simulink model "CSTRExampleLinear"  (R2020a)
settings: Solver=FixedStepAuto  StartTime=0.0  StopTime=6  FixedStep=10e-3  MaxStep=10e-3  RelTol=1e-3
InitFcn:
  | CSTRInit;
values from neighbouring files (symbols this model uses):
  A = [-Fr0/V-k1-2*k3*Ca0, 0; k1, -Fr0/V-k2]    [CSTRInit.m]
  B = [6.341719*(Cai0-Ca0)/V, Fr0/V; -6.341719*Cb0/V, 0]    [CSTRInit.m]
  C = [0 100/1.5714]    [CSTRInit.m]
  Ca0 = 2.917496611031752    (= 2.91749661103)    [CSTRComputeOP.m]    (also in CSTRInit.m)
  Cai0 = 10    [CSTRInit.m]
  Cb0 = 1.099991103606458    (= 1.09999110361)    [CSTRComputeOP.m]    (also in CSTRInit.m)
  D = [0, 0]    [CSTRInit.m]
  k1 = 5/6    (= 0.833333333333)    [CSTRComputeOP.m]    (also in CSTRInit.m; CSTROP.m = param(1); sfun_CSTR.m = param(1))
  k2 = 5/3    (= 1.66666666667)    [CSTRComputeOP.m]    (also in CSTRInit.m; CSTROP.m = param(2); sfun_CSTR.m = param(2))
  k3 = 1/6    (= 0.166666666667)    [CSTRComputeOP.m]    (also in CSTRInit.m; CSTROP.m = param(3); sfun_CSTR.m = param(3))
  u0 = 60    [CSTRInit.m]
  V = 700    [CSTRComputeOP.m]    (also in CSTRInit.m; CSTROP.m = param(4); sfun_CSTR.m = param(4))
  y0 = 100/1.5714*Cb0    (= 70.000706606)    [CSTRInit.m]
settings Model: Creator=david  LastModifiedBy=david

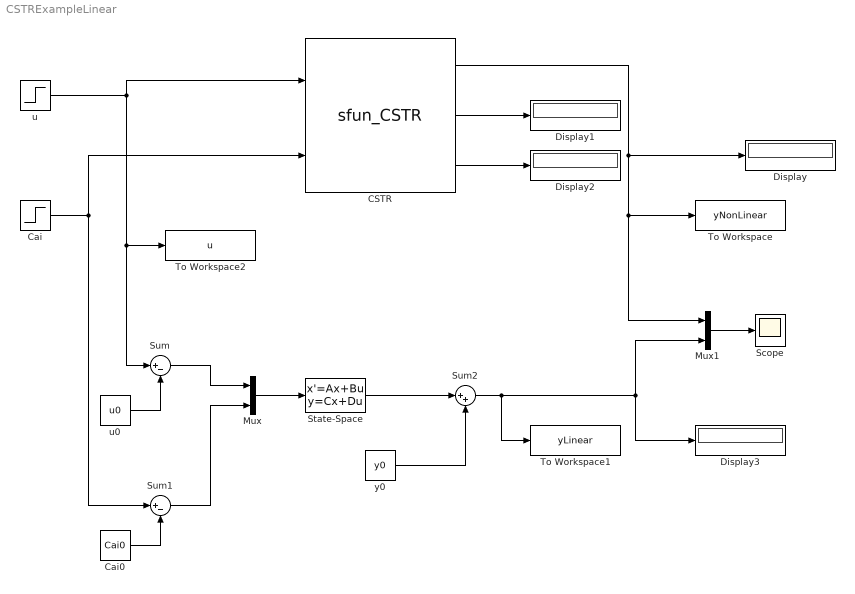
== system CSTRExampleLinear ==
  CSTR : M-S-Function  FunctionName=sfun_CSTR  Parameters=|  mask{k1=k1, k2=k2, k3=k3, V=V, Ca0=Ca0, Cb0=Cb0}
      | [k1;
      | k2;
      | k3; V], [Ca0; Cb0]
      mask Display:
      | port_label('output', 1, 'y')
      | port_label('output', 2, 'Ca')
      | port_label('output', 3, 'Cb')
      | port_label('input', 1, 'u')
      | port_label('input', 2, 'Cai')
      | image('VandeVusse.png')
  Cai : Step  Time=20  Before=10  After=10  SampleTime=0
  Cai0 : Constant  Value=Cai0
  Display{,1..3} (4 alike) : Display
  Mux : Mux  Inputs=2
  Mux1 : Mux  Inputs=2
  Scope : Scope
  State-Space : StateSpace  A=A  B=B  C=C  D=D  InitialCondition=0
  Sum : Sum  Inputs=|+-
  Sum1 : Sum  Inputs=|+-
  Sum2 : Sum  Inputs=|++
  To Workspace : ToWorkspace  VariableName=yNonLinear  SaveFormat=Timeseries  SampleTime=-1
  To Workspace1 : ToWorkspace  VariableName=yLinear  SaveFormat=Timeseries  SampleTime=-1
  To Workspace2 : ToWorkspace  VariableName=u  SaveFormat=Timeseries  SampleTime=-1
  u : Step  Time=0  Before=60  After=65  SampleTime=0
  u0 : Constant  Value=u0
  y0 : Constant  Value=y0
  wires:
  CSTR/1 -> To Workspace/1, Mux1/1, Display/1
  Cai/1 -> Sum1/1, CSTR/2
  u0/1 -> Sum/2
  Cai0/1 -> Sum1/2
  Sum/1 -> Mux/1
  Sum1/1 -> Mux/2
  Mux/1 -> State-Space/1
  y0/1 -> Sum2/2
  Sum2/1 -> To Workspace1/1, Display3/1, Mux1/2
  Mux1/1 -> Scope/1
  CSTR/2 -> Display1/1
  CSTR/3 -> Display2/1
  State-Space/1 -> Sum2/1
  u/1 -> To Workspace2/1, Sum/1, CSTR/1
